simulink model "Simulink_compensador_adelanto"  (Simulink 8.1)
settings: Solver=ode45  StartTime=0.0  StopTime=3e-3  RelTol=1e-3
values from neighbouring files (symbols this model uses):
  den_G2 = R21    (= 10000)    [tp11.m]
  den_G3 = [1 (R32*C31+R31*C31)/(R31*R32*C31*C32) 1/(R31*R32*C31*C32)]    [tp11.m]
  num_G2 = R21+R22    (= 66000)    [tp11.m]
  num_G3 = 1/(R31*R32*C31*C32)    (= 5275931.20186)    [tp11.m]
undefined symbols (not defined in the file or in its folder): den_ca, den_la, num_ca, num_la
settings Model: Creator=alumno  LastModifiedBy=CLA
settings DebuggingCC: SolverPrmCheckMsg=none  FcnCallInpInsideContextMsg=EnableAllAsWarning
settings SFSimCC: SimUserSources=C:\MATLAB2012aPortable  SimUserIncludeDirs=C:\MATLAB2012aPortable  SimUserLibraries=C:\MATLAB2012aPortable
settings GRTTargetCC: CombineOutputUpdateFcns=on  GRTInterface=off

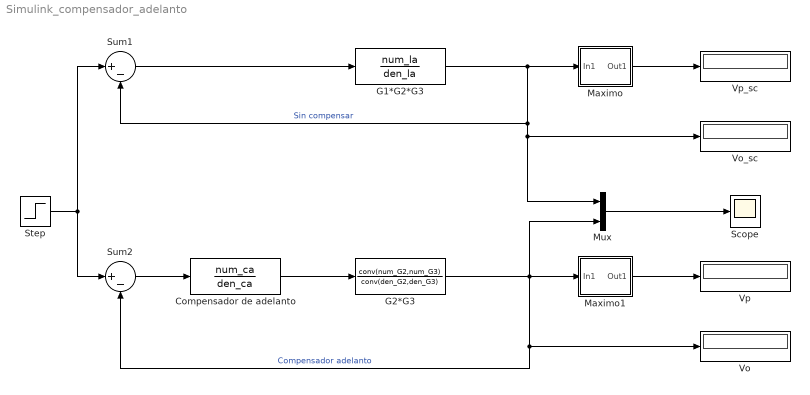
== system Simulink_compensador_adelanto ==
  Compensador de adelanto : TransferFcn  Numerator=num_ca  Denominator=den_ca
  G1*G2*G3 : TransferFcn  Numerator=num_la  Denominator=den_la
  G2*G3 : TransferFcn  Numerator=conv(num_G2,num_G3)  Denominator=conv(den_G2,den_G3)
  "Maximo " : Subsystem
  Maximo1 : Subsystem
  Mux : Mux  Inputs=2
  Scope : Scope
      settings: ShowLegends=on  TimeRange=0.003  YMin=0  YMax=1.4  SaveName=OUT
  Step : Step  Time=0  SampleTime=0
  Sum1 : Sum  Inputs=|+-
  Sum2 : Sum  Inputs=|+-
  Vo : Display
  Vo_sc : Display
  Vp : Display
  Vp_sc : Display
  wires:
  Sum2/1 -> Compensador de adelanto/1
  G2*G3/1 -> Maximo1/1(In1), Mux/2, Vo/1, Sum2/2  "Compensador adelanto"
  Sum1/1 -> G1*G2*G3/1
  Step/1 -> Sum2/1, Sum1/1
  Compensador de adelanto/1 -> G2*G3/1
  G1*G2*G3/1 -> "Maximo "/1(In1), Vo_sc/1, Mux/1, Sum1/2  "Sin compensar"
  Mux/1 -> Scope/1
  Maximo1/1(Out1) -> Vp/1
  "Maximo "/1(Out1) -> Vp_sc/1

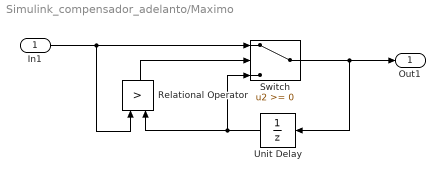
== system Simulink_compensador_adelanto/Maximo  ==
  In1 : Inport
  Relational Operator : RelationalOperator  Operator=>  OutDataTypeStr=boolean
  Switch : Switch
  Unit Delay : UnitDelay  SampleTime=-1
  Out1 : Outport
  wires:
  In1/1 -> Relational Operator/1, Switch/1
  Unit Delay/1 -> Relational Operator/2, Switch/3
  Relational Operator/1 -> Switch/2
  Switch/1 -> Unit Delay/1, Out1/1

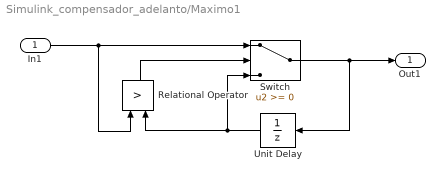
== system Simulink_compensador_adelanto/Maximo1 ==
  In1 : Inport
  Relational Operator : RelationalOperator  Operator=>  OutDataTypeStr=boolean
  Switch : Switch
  Unit Delay : UnitDelay  SampleTime=-1
  Out1 : Outport
  wires:
  In1/1 -> Relational Operator/1, Switch/1
  Unit Delay/1 -> Relational Operator/2, Switch/3
  Relational Operator/1 -> Switch/2
  Switch/1 -> Unit Delay/1, Out1/1
